simulink library "GPS_time_prop_lib"  (R2016b)
settings: Solver=VariableStepAuto  StartTime=0.0  StopTime=10.0  RelTol=1e-3
settings Model: Creator=Taylor  LastModifiedBy=Taylor

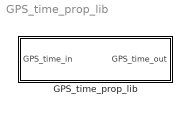
== system GPS_time_prop_lib ==
  GPS_time_prop_lib : Subsystem

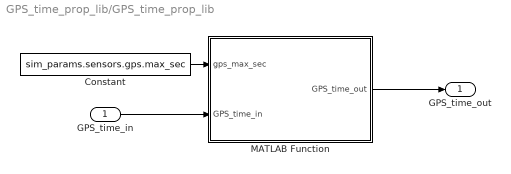
== system GPS_time_prop_lib/GPS_time_prop_lib ==
  GPS_time_in : Inport
  Constant : Constant  Value=sim_params.sensors.gps.max_sec
  MATLAB Function : MATLAB Function  TreatAsAtomicUnit=on
  GPS_time_out : Outport
  wires:
  MATLAB Function/1(GPS_time_out) -> GPS_time_out/1
  GPS_time_in/1 -> MATLAB Function/2(GPS_time_in)
  Constant/1 -> MATLAB Function/1(gps_max_sec)

== matlab function GPS_time_prop_lib/MATLAB Function ==
  data: gps_max_sec input; GPS_time_out output; GPS_time_in input
function GPS_time_out  = fcn(gps_max_sec,GPS_time_in)

gps_sec     = GPS_time_in(1);
gps_week    = GPS_time_in(2);

if( mod(gps_sec,gps_max_sec) == 0 && gps_sec ~= 0 )
    gps_week = gps_week + 1;
    gps_sec = gps_sec - gps_max_sec;
else
    gps_sec = gps_sec + 1;
    gps_week = gps_week;
end

GPS_time_out    = [ gps_sec; gps_week ];
